simulink model "nsdynamic_Force3"  (R2021b)
settings: Solver=ode4  StartTime=0.0  StopTime=10.0  RelTol=1e-3
InitFcn:
  | initialization
undefined symbols (not defined in the file or in its folder): dynNS_Force3, trajectory
settings Model: Creator=AzamaoZ  LastModifiedBy=AzamaoZ

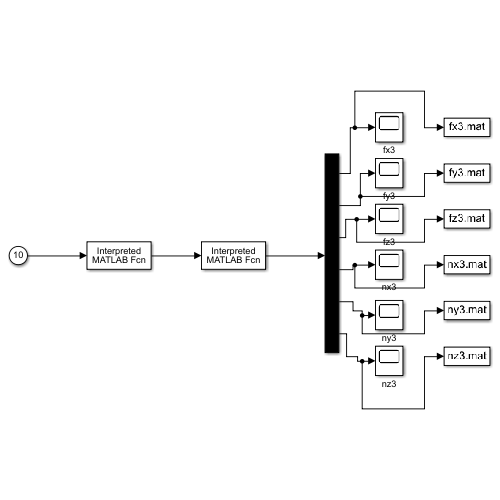
[thumbnail: Simulink's stored preview of the top-level diagram]
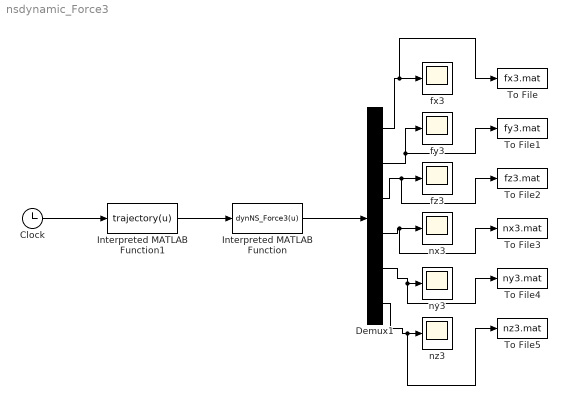
== system nsdynamic_Force3 ==
  Clock : Clock
  Demux1 : Demux  Outputs=6
  Interpreted MATLAB Function : MATLABFcn  MATLABFcn=dynNS_Force3(u)  OutputDimensions=6
  Interpreted MATLAB Function1 : MATLABFcn  MATLABFcn=trajectory(u)
  To File : ToFile  Filename=fx3.mat  MatrixName=fx3  SaveFormat=Timeseries
  To File1 : ToFile  Filename=fy3.mat  MatrixName=fy3  SaveFormat=Timeseries
  To File2 : ToFile  Filename=fz3.mat  MatrixName=fz3  SaveFormat=Timeseries
  To File3 : ToFile  Filename=nx3.mat  MatrixName=nx3  SaveFormat=Timeseries
  To File4 : ToFile  Filename=ny3.mat  MatrixName=ny3  SaveFormat=Timeseries
  To File5 : ToFile  Filename=nz3.mat  MatrixName=nz3  SaveFormat=Timeseries
  fx3 : Scope
  fy3 : Scope
  fz3 : Scope
  nx3 : Scope
  ny3 : Scope
  nz3 : Scope
  wires:
  Interpreted MATLAB Function/1 -> Demux1/1
  Clock/1 -> Interpreted MATLAB Function1/1
  Demux1/2 -> fy3/1, To File1/1
  Demux1/4 -> To File3/1, nx3/1
  Demux1/6 -> To File5/1, nz3/1
  Demux1/5 -> To File4/1, ny3/1
  Demux1/3 -> To File2/1, fz3/1
  Interpreted MATLAB Function1/1 -> Interpreted MATLAB Function/1
  Demux1/1 -> To File/1, fx3/1
